simulink model "lavagna"  (R2020b)
settings: Solver=VariableStepAuto  StartTime=0.0  StopTime=10.0  RelTol=1e-3
settings Model: Creator=marco  LastModifiedBy=marco

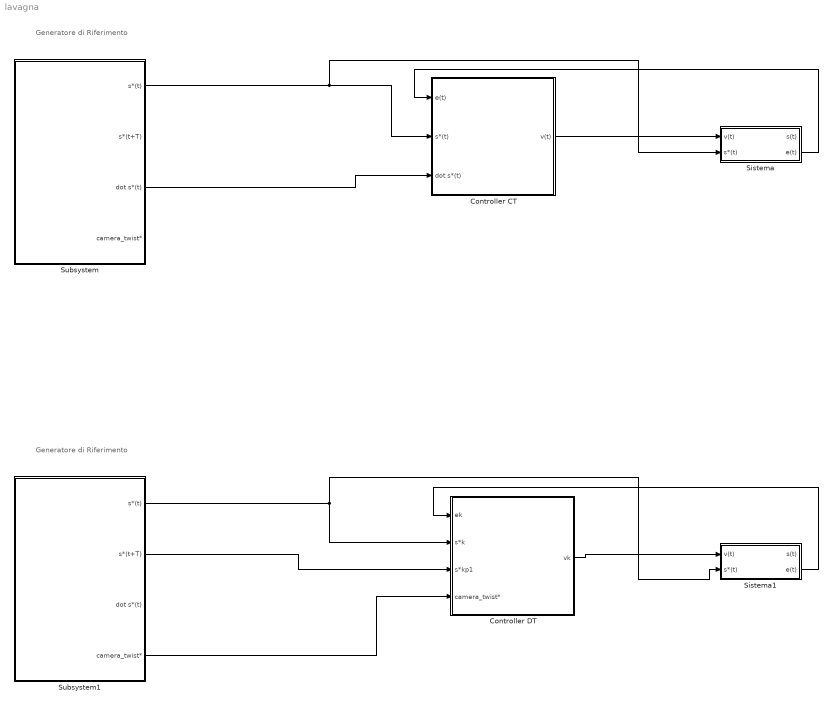
== system lavagna ==
  note: Generatore di Riferimento
  note: Generatore di Riferimento
  Controller CT : Subsystem
  Controller DT : Subsystem
  Sistema : Subsystem
  Sistema1 : Subsystem
  Subsystem : Subsystem
  Subsystem1 : Subsystem
  wires:
  Subsystem/3(dot s*(t)) -> Controller CT/3(dot s*(t))
  Subsystem/1(s*(t)) -> Sistema/2(s*(t)), Controller CT/2(s*(t))
  Controller CT/1(v(t)) -> Sistema/1(v(t))
  Sistema/2(e(t)) -> Controller CT/1(e(t))
  Controller DT/1(vk) -> Sistema1/1(v(t))
  Sistema1/2(e(t)) -> Controller DT/1(ek)
  Subsystem1/1(s*(t)) -> Controller DT/2(s*k), Sistema1/2(s*(t))
  Subsystem1/4(camera_twist*) -> Controller DT/4(camera_twist*)
  Subsystem1/2(s*(t+T)) -> Controller DT/3(s*kp1)

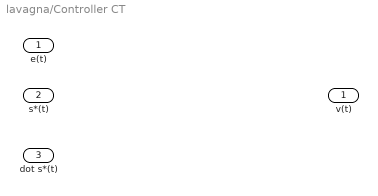
== system lavagna/Controller CT ==
  e(t) : Inport
  s*(t) : Inport  Port=2
  dot s*(t) : Inport  Port=3
  v(t) : Outport

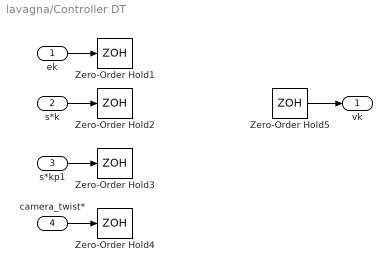
== system lavagna/Controller DT ==
  ek : Inport
  s*k : Inport  Port=2
  s*kp1 : Inport  Port=3
  camera_twist* : Inport  Port=4
  Zero-Order Hold{1..5} (5 alike) : ZeroOrderHold  SampleTime=-1
  vk : Outport
  wires:
  ek/1 -> Zero-Order Hold1/1
  s*k/1 -> Zero-Order Hold2/1
  s*kp1/1 -> Zero-Order Hold3/1
  camera_twist*/1 -> Zero-Order Hold4/1
  Zero-Order Hold5/1 -> vk/1

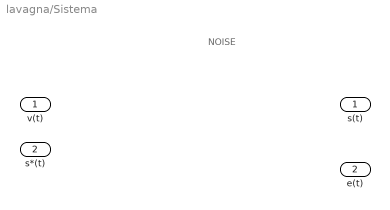
== system lavagna/Sistema ==
  note: NOISE
  v(t) : Inport
  s*(t) : Inport  Port=2
  s(t) : Outport
  e(t) : Outport  Port=2

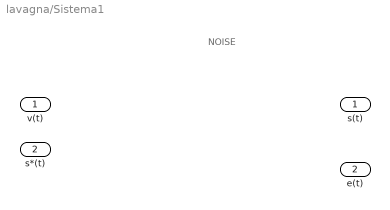
== system lavagna/Sistema1 ==
  note: NOISE
  v(t) : Inport
  s*(t) : Inport  Port=2
  s(t) : Outport
  e(t) : Outport  Port=2

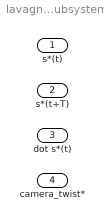
== system lavagna/Subsystem ==
  s*(t) : Outport
  s*(t+T) : Outport  Port=2
  dot s*(t) : Outport  Port=3
  camera_twist* : Outport  Port=4

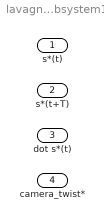
== system lavagna/Subsystem1 ==
  s*(t) : Outport
  s*(t+T) : Outport  Port=2
  dot s*(t) : Outport  Port=3
  camera_twist* : Outport  Port=4
